simulink model "Schmitt"  (R2026a)
settings: Solver=VariableStepAuto  StartTime=75  StopTime=100
model workspace (MAT data in the model file):
  x = 3000
libraries: fl_lib x3, nesl_utility x3, ee_lib x1
settings Model: Creator=Next  LastModifiedBy=Next

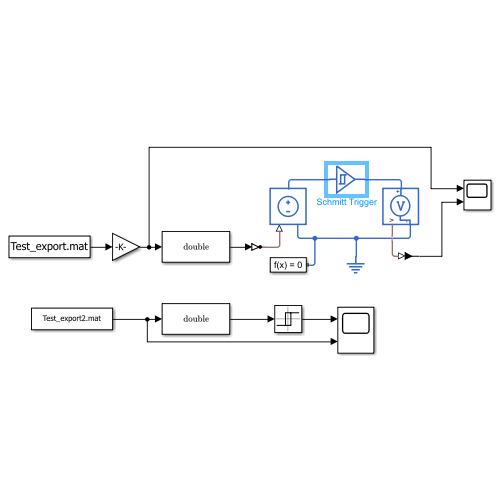
[thumbnail: Simulink's stored preview of the top-level diagram]
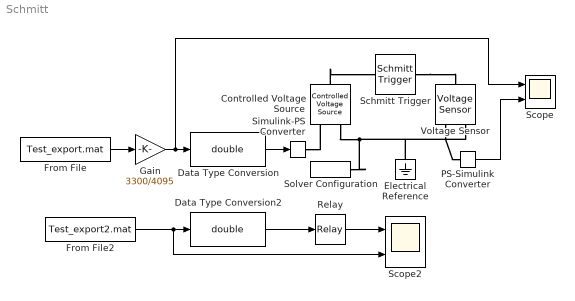
== system Schmitt ==
  Controlled Voltage Source : fl_lib/Electrical/Electrical Sources/Controlled Voltage Source
  Data Type Conversion : DataTypeConversion  OutDataTypeStr=double  SaturateOnIntegerOverflow=off  RndMeth=Floor
  Data Type Conversion2 : DataTypeConversion  OutDataTypeStr=double  SaturateOnIntegerOverflow=off  RndMeth=Floor
  Electrical Reference : fl_lib/Electrical/Electrical Elements/Electrical Reference
  From File : FromFile  FileName=Test_export.mat  SampleTime=0
  From File2 : FromFile  FileName=Test_export2.mat  SampleTime=0
  Gain : Gain  Gain=3300/4095
  PS-Simulink Converter : nesl_utility/PS-Simulink Converter  PhysicalDomain=network_engine_domain  SubClassName=ps_output  LeftPortType=input  RightPortType=output  PseudoPeriodic=off  Frequencies=[]  VectorFormat=inherit  Unit=inherit  AffineConversion=off
  Relay : Relay  OnSwitchValue=3000  OffSwitchValue=1000  OnOutputValue=5000
  Schmitt Trigger : ee_lib/Integrated Circuits/Logic/Schmitt Trigger  V_IL=1.1 kV  V_IH=2.2 kV  C_IN=5 pF  output_type=ee.enum.ic.outputType.linear  V_OL=0 kV  V_OH=5 kV  V_CC=5 V  V_meas=5 V  R_OUT=25 Ohm  R_OH=[25, 250] Ohm  I_OH=63 mA  R_OL=[30, 800] Ohm  I_OL=-45 mA  Delay=25 ns  Ron=5 Ohm  Vf=0.6 V  output_state=ee.enum.ic.initialState.low
  Scope : Scope  NumInputPorts=2
      settings: ActiveDisplayYMinimum=-773.73803092783874  ActiveDisplayYMaximum=5611.6013695275042
  Scope2 : Scope  NumInputPorts=2
      settings: ActiveDisplayYMinimum=-1817.6759189734721  ActiveDisplayYMaximum=6245.0739403107837  DataLoggingVariableName=ScopeData2
  Simulink-PS Converter : nesl_utility/Simulink-PS Converter  PhysicalDomain=network_engine_domain  SubClassName=ps_input  LeftPortType=input  RightPortType=output  PseudoPeriodic=off  Frequencies=[]  NoiseDistribution=none  NoiseParameters=[]  Unit=1  AffineConversion=off  FilteringAndDerivatives=filter  SimscapeFilterOrder=1  InputFilterTimeConstant=0.001  UdotUserProvided=0
  Solver Configuration : nesl_utility/Solver Configuration  PhysicalDomain=network_engine_domain  SubClassName=solver  LeftPortType=input  RightPortType=generic  Tones=[]  Harmonics=[]  SimulateNoise=off  Profile=off  UseLocalSampling=off  EnableSwitchedLinearOptims=on  FrequencyDomain=off  UseCCode=off  RelTol=0.001  AbsTol=0.001  MinStep=1e-09  ToWorkspace=off  RevertToSquareIcSolve=off  NumHomotopyIterations=100  PhasorMode=off  PhasorModeNumHarmonics=1  ConsistencySolver=NEWTON_XTOL_AFTER_FTOL  CanonicalOrdering=CANONICAL  OptimizeIntermediates=OPTIMIZED  IndexReductionMethod=DerivativeReplacement  DoDC=off  ResidualTolerance=1e-09  ConsistencyTolSource=GLOBAL  ConsistencyAbsTol=0.001  ConsistencyRelTol=0.001  ConsistencyTolFactor=0.001  UseLocalSolver=on  LocalSolverChoice=NE_BACKWARD_EULER_ADVANCER  ResolveIndetEquations=on  FunctionEvalNumThread=1  LocalSolverSampleTime=0.001  DoFixedCost=off  MaxNonlinIter=3  MaxModeIter=2  ComputeImpulses=off  ImpulseIterations=2  LinearAlgebra=auto  LinearAlgebraNumThread=0  EquationFormulation=NE_TIME_EF  DelaysMemoryBudget=1024  AutomaticFiltering=on  FilteringTimeConstant=0.001  PartitionStorageMethod=AS_NEEDED  PartitionMemoryBudget=1024  PartitionMethod=ROBUST  MultibodyUseLocalSolver=off  MultibodyLocalSolverChoice=ODE1  MultibodyLocalSolverSampleTime=0.001
  Voltage Sensor : fl_lib/Electrical/Electrical Sensors/Voltage Sensor
  wires:
  Data Type Conversion/1 -> Simulink-PS Converter/1
  PS-Simulink Converter/1 -> Scope/2
  From File2/1 -> Scope2/2, Data Type Conversion2/1
  Data Type Conversion2/1 -> Relay/1
  Relay/1 -> Scope2/1
  Gain/1 -> Scope/1, Data Type Conversion/1
  From File/1 -> Gain/1
  connections:
  Simulink-PS Converter/RConn1 -- Controlled Voltage Source/RConn1
  Controlled Voltage Source/RConn2 -- Solver Configuration/RConn1 -- Voltage Sensor/RConn2 -- Electrical Reference/LConn1
  Controlled Voltage Source/LConn1 -- Schmitt Trigger/LConn1
  Voltage Sensor/RConn1 -- PS-Simulink Converter/LConn1
  Schmitt Trigger/RConn1 -- Voltage Sensor/LConn1
